simulink model "model"  (R2020a)
settings: Solver=ode3  StartTime=0.0  StopTime=50  FixedStep=0.001  RelTol=1e-3
values from neighbouring files (symbols this model uses):
  K = DesiredLoop/tfCar    [main_a34_loop_shaping.m]
undefined symbols (not defined in the file or in its folder): sigbuilder_block
settings Model: Creator=Daniel  LastModifiedBy=Daniel

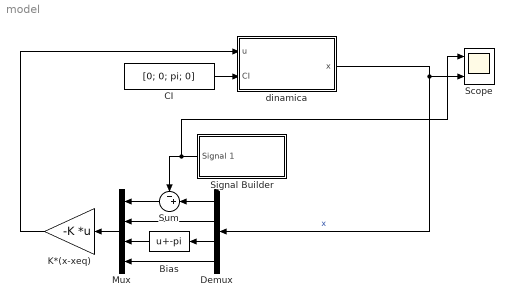
== system model ==
  Bias : Bias  Bias=-pi
  CI : Constant  Value=[0; 0; pi; 0]
  Demux : Demux
  K*(x-xeq) : Gain  Gain=-K  Multiplication=Matrix(K*u)
  Mux : Mux
  Scope : Scope  NumInputPorts=2
  Signal Builder : Subsystem  Tag=STV Subsys  LoadFcn=sigbuilder_block('load');  StartFcn=sigbuilder_block('start');  StopFcn=sigbuilder_block('stop');  ClipboardFcn=sigbuilder_block('clipboard');  mask(Sigbuilder block){tuvar=[0:10]}
      mask help: Simulink:masks:SigbuilderBlock_MD
      mask init:
      | if ~strcmp(get_param(bdroot(gcbh),'SimulationStatus'),'stopped') tuvar = sigbuilder_block('maskInit'); end
      settings: CopyFcn=sigbuilder_block('copy');  DeleteFcn=sigbuilder_block('delete');  ModelCloseFcn=sigbuilder_block('modelClose');  PreSaveFcn=sigbuilder_block('preSave');  PauseFcn=sigbuilder_block('pause');  ContinueFcn=sigbuilder_block('continue');  NameChangeFcn=sigbuilder_block('namechange');  OpenFcn=sigbuilder_block('open',[245.25 404.25 550.5 296.25 ]);  CloseFcn=sigbuilder_block('close');
      mask Display: plot(0, 0, 100, 100,[2, 2, 32, 32, 2], [68, 8, 8, 68, 68],[32, 2], [38, 38], [32, 19, 2],[53, 60, 44], [32, 17, 17, 2],[16, 16, 31, 31]);txt = getActiveGroup(gcbh);text(2, 100, txt,'verticalAlignment', 'top');
  Sum : Sum  Inputs=-+|
  dinamica : Subsystem
  wires:
  Mux/1 -> K*(x-xeq)/1
  Sum/1 -> Mux/1
  Demux/2 -> Mux/2
  Demux/4 -> Mux/4
  Demux/3 -> Bias/1
  Demux/1 -> Sum/2
  Signal Builder/1(Signal 1) -> Scope/1, Sum/1
  dinamica/1(x) -> Demux/1, Scope/2  "x"
  CI/1 -> dinamica/2(CI)
  K*(x-xeq)/1 -> dinamica/1(u)
  Bias/1 -> Mux/3

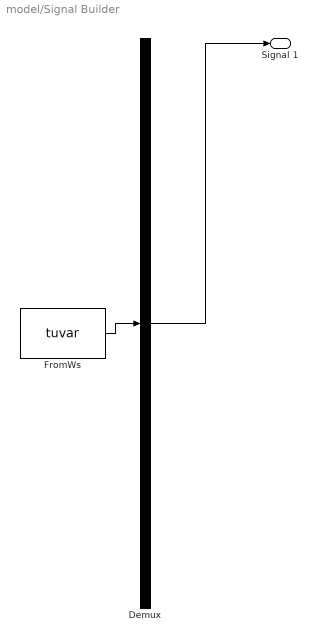
== system model/Signal Builder ==
  Demux : Demux  Tag=STV Demux  Outputs=1
      settings: DisplayOption=none
  FromWs : FromWorkspace  Tag=STV FromWs  VariableName=tuvar
      SigBuilderData=|
      | common.afterFinalStr = 'Extrapolate'
      | common.sampleTime = 0
      | dataSet.timeRange = [0 50]
      | dataSet.name = 'Group 1'
      | sbobj.Groups.Name = 'Group 1'
      | sbobj.Groups.Signals.Name = 'Signal 1'
      | sbobj.Groups.Signals.XData = [0 4 4 11.2 11.2 16 16 22.8 22.8 32.8 32.8 43.1 43.1 50]
      | sbobj.Groups.Signals.YData = [0 0 0.41 0.41 0.6 0.6 0.32 0.32 0.8 0.8 0.6 0.6 0 0]
      | sbobj.Groups.TimeRange = [0 50]
  Signal 1 : Outport  Tag=STV Outport
  wires:
  Demux/1 -> Signal 1/1
  FromWs/1 -> Demux/1

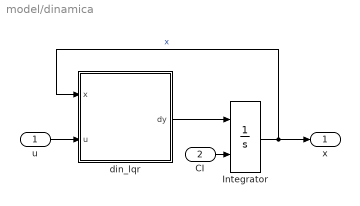
== system model/dinamica ==
  u : Inport
  CI : Inport  Port=2
  Integrator : Integrator  InitialConditionSource=external  InitialCondition=[0; 0; pi + 0.01; 0]
  din_lqr : MATLAB Function  TreatAsAtomicUnit=on
  x : Outport
  wires:
  din_lqr/1(dy) -> Integrator/1
  Integrator/1 -> x/1, din_lqr/1(x)  "x"
  u/1 -> din_lqr/2(u)
  CI/1 -> Integrator/2

== matlab function model/dinamica/din_lqr ==
  data: x input; u input; dy output
function dy = carropend(x, u)
    % carac. modelo
    m = 1.0;
    M = 5.0;
    L = 2.0;
    g = -10.0;
    d = 1.0;
    
    % equ. diferencial
    dy = fn_eq_diferencial(x,m,M,L,g,d,u);
